simulink model "Am"  (R2023b)
settings: Solver=VariableStepAuto  StartTime=0.0  StopTime=5  RelTol=1e-3
settings Model: Creator=HP  LastModifiedBy=HP

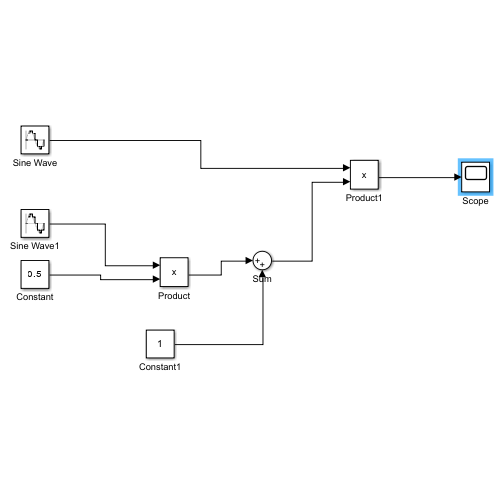
[thumbnail: Simulink's stored preview of the top-level diagram]
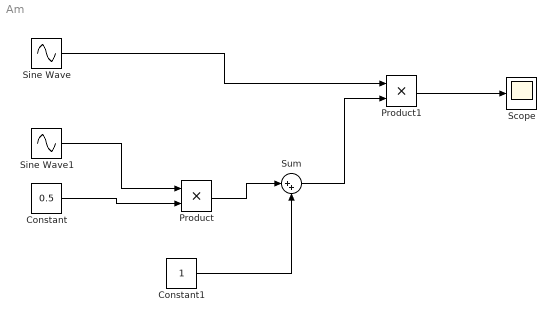
== system Am ==
  Constant : Constant  Value=0.5
  Constant1 : Constant
  Product : Product
  Product1 : Product
  Scope : Scope
  Sine Wave : Sin  Frequency=2*pi*25  SampleTime=1/5000
  Sine Wave1 : Sin  Frequency=2*pi  SampleTime=1/5000
  Sum : Sum  Inputs=|++
  wires:
  Sine Wave/1 -> Product1/1
  Sine Wave1/1 -> Product/1
  Constant/1 -> Product/2
  Constant1/1 -> Sum/2
  Product/1 -> Sum/1
  Sum/1 -> Product1/2
  Product1/1 -> Scope/1
